simulink model "Pedirtiempo_Harness6"  (R2020b)
settings: Solver=VariableStepAuto  StartTime=0.0  StopTime=10.0  RelTol=1e-3
settings Model: Creator=cacha  LastModifiedBy=cacha

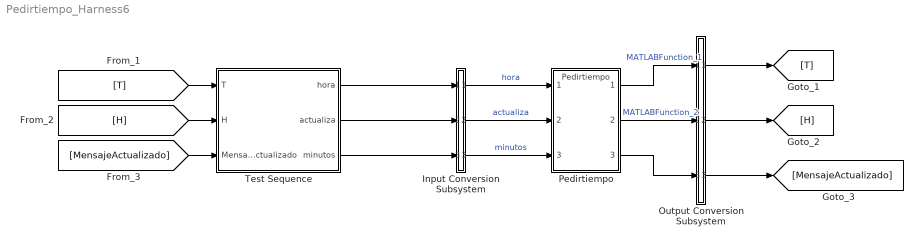
== system Pedirtiempo_Harness6 ==
  Input Conversion Subsystem : Subsystem  Tag=__SLT_ICS__  Description=|
      | Signal spec.
      | and routing
      settings: AttributesFormatString=%<Description>
  Output Conversion Subsystem : Subsystem  Tag=__SLT_OCS__  Description=|
      | Signal spec.
      | and routing
      settings: AttributesFormatString=%<Description>
  Pedirtiempo : ModelReference  ModelNameDialog=Pedirtiempo  SimulationMode=Normal  ModelReferenceVersion=1.31
  Test Sequence : Test Sequence  TreatAsAtomicUnit=on
  wires:
  Test Sequence/1(hora) -> Input Conversion Subsystem/1(Inport_1)
  Test Sequence/2(actualiza) -> Input Conversion Subsystem/2(Inport_2)
  Test Sequence/3(minutos) -> Input Conversion Subsystem/3(Inport_3)
  [T] -> Test Sequence/1(T)
  [H] -> Test Sequence/2(H)
  [MensajeActualizado] -> Test Sequence/3(MensajeActualizado)
  Output Conversion Subsystem/1(Outport_1) -> [T]
  Output Conversion Subsystem/2(Outport_2) -> [H]
  Output Conversion Subsystem/3(Outport_3) -> [MensajeActualizado]
  Input Conversion Subsystem/1(Outport_1) -> Pedirtiempo/1  "hora"
  Input Conversion Subsystem/2(Outport_2) -> Pedirtiempo/2  "actualiza"
  Input Conversion Subsystem/3(Outport_3) -> Pedirtiempo/3  "minutos"
  Pedirtiempo/1 -> Output Conversion Subsystem/1(Inport_1)  "MATLABFunction_1"
  Pedirtiempo/2 -> Output Conversion Subsystem/2(Inport_2)  "MATLABFunction_2"
  Pedirtiempo/3 -> Output Conversion Subsystem/3(Inport_3)

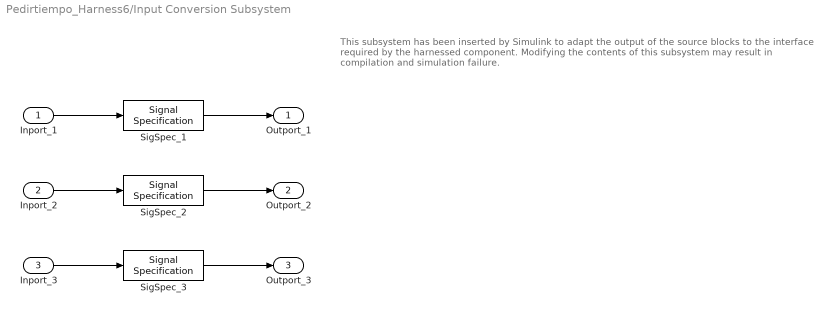
== system Pedirtiempo_Harness6/Input Conversion Subsystem ==
  note: This subsystem has been inserted by Simulink to adapt the output of the source blocks to the interface required by the harnessed component.
      |  Modifying the contents of this subsystem may result in compilation and simulation failure.
  Inport_1 : Inport
  Inport_2 : Inport  Port=2
  Inport_3 : Inport  Port=3
  SigSpec_1 : SignalSpecification  OutDataTypeStr=double  Dimensions=[1]  SampleTime=[-1, 0]
  SigSpec_2 : SignalSpecification  OutDataTypeStr=double  Dimensions=[1]  SampleTime=[-1, 0]
  SigSpec_3 : SignalSpecification  OutDataTypeStr=double  Dimensions=[1]  SampleTime=[-1, 0]
  Outport_1 : Outport
  Outport_2 : Outport  Port=2
  Outport_3 : Outport  Port=3
  wires:
  SigSpec_1/1 -> Outport_1/1
  Inport_1/1 -> SigSpec_1/1
  SigSpec_2/1 -> Outport_2/1
  Inport_2/1 -> SigSpec_2/1
  SigSpec_3/1 -> Outport_3/1
  Inport_3/1 -> SigSpec_3/1

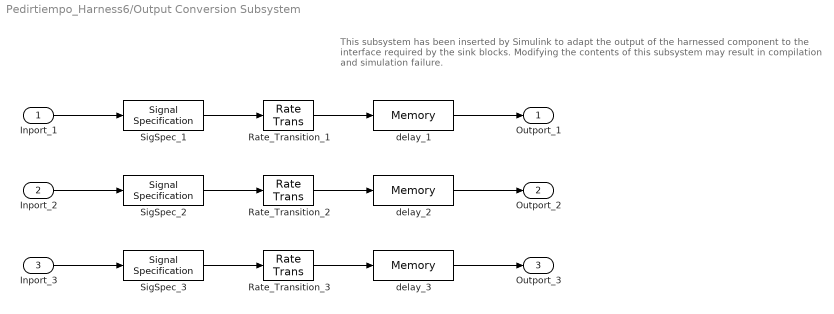
== system Pedirtiempo_Harness6/Output Conversion Subsystem ==
  note: This subsystem has been inserted by Simulink to adapt the output of the harnessed component to the interface required by the sink blocks.
      |  Modifying the contents of this subsystem may result in compilation and simulation failure.
  Inport_1 : Inport
  Inport_2 : Inport  Port=2
  Inport_3 : Inport  Port=3
  Rate_Transition_1 : RateTransition  OutPortSampleTimeOpt=Inherit
  Rate_Transition_2 : RateTransition  OutPortSampleTimeOpt=Inherit
  Rate_Transition_3 : RateTransition  OutPortSampleTimeOpt=Inherit
  SigSpec_1 : SignalSpecification  OutDataTypeStr=double  Dimensions=[1]
  SigSpec_2 : SignalSpecification  OutDataTypeStr=double  Dimensions=[1]
  SigSpec_3 : SignalSpecification  OutDataTypeStr=double  Dimensions=[1]
  delay_1 : Memory
  delay_2 : Memory
  delay_3 : Memory
  Outport_1 : Outport
  Outport_2 : Outport  Port=2
  Outport_3 : Outport  Port=3
  wires:
  Inport_1/1 -> SigSpec_1/1
  SigSpec_1/1 -> Rate_Transition_1/1
  Rate_Transition_1/1 -> delay_1/1
  delay_1/1 -> Outport_1/1
  Inport_2/1 -> SigSpec_2/1
  SigSpec_2/1 -> Rate_Transition_2/1
  Rate_Transition_2/1 -> delay_2/1
  delay_2/1 -> Outport_2/1
  Inport_3/1 -> SigSpec_3/1
  SigSpec_3/1 -> Rate_Transition_3/1
  Rate_Transition_3/1 -> delay_3/1
  delay_3/1 -> Outport_3/1

== stateflow chart Pedirtiempo_Harness6/Test Sequence ==
  settings: stateMachineType=SIMPLIFIED_MACHINE
  state Run
    %% Initialize data outputs.
    hora = 0;
    actualiza = 0;
    minutos = 0;
    settings: description=Se simula que pasa media hora
  state step_1
    hora=0;
    actualiza=0;
    minutos=30;
    settings: description=Una vez sucede actualizamos
  state step_2
    hora=0;
    actualiza=0;
    minutos=0;
    settings: description=Se simula que pasa un día
  state step_3
    hora=24;
    actualiza=0;
    minutos=0;
    settings: description=Una vez sucede actualizamos
  state step_4
    hora=0;
    actualiza=0;
    minutos=0;
    settings: description=Se simula que el usuario decide actualizar
  state step_5
    hora=0;
    actualiza=1;
    minutos=0;
    settings: description=Actualizamos
  state step_6
    hora=0;
    actualiza=0;
    minutos=0;
  (default) -> Run
  Run -> step_1 : [
      | after(2,sec)
      | ]
  step_1 -> step_2 : [
      | true
      | ]
  step_2 -> step_3 : [
      | after(4,sec)
      | ]
  step_3 -> step_4 : [
      | true
      | ]
  step_4 -> step_5 : [
      | after(1,sec)
      | ]
  step_5 -> step_6 : [
      | true
      | ]
  data: T input double size=[1]; H input double size=[1]; MensajeActualizado input double size=[1]; hora output double size=[1]; actualiza output double size=[1]; minutos output double size=[1]
